simulink model "simulare_regulator_discret_etapa1"  (R2020a)
settings: Solver=VariableStepAuto  StartTime=0.0  StopTime=500  RelTol=1e-3
settings Model: Creator=user  LastModifiedBy=user

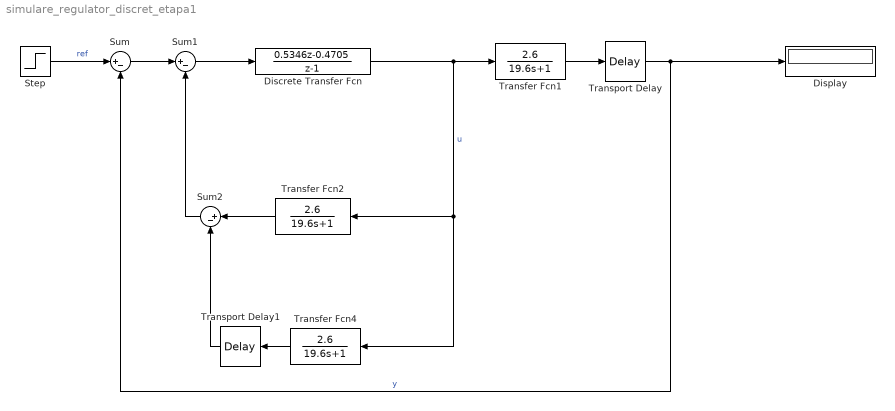
== system simulare_regulator_discret_etapa1 ==
  Discrete Transfer Fcn : DiscreteTransferFcn  Numerator=[0.5346 -0.4705]  Denominator=[1 -1]  SampleTime=2.5
  Display : Display
  Step : Step  SampleTime=2.5
  Sum : Sum  Inputs=|+-
  Sum1 : Sum  Inputs=|+-
  Sum2 : Sum  Inputs=|+-
  Transfer Fcn1 : TransferFcn  Numerator=[2.6]  Denominator=[19.6 1]
  Transfer Fcn2 : TransferFcn  Numerator=[2.6]  Denominator=[19.6 1]
  Transfer Fcn4 : TransferFcn  Numerator=[2.6]  Denominator=[19.6 1]
  Transport Delay : TransportDelay  DelayTime=5
  Transport Delay1 : TransportDelay  DelayTime=5
  wires:
  Transport Delay1/1 -> Sum2/2
  Sum2/1 -> Sum1/2
  Transfer Fcn4/1 -> Transport Delay1/1
  Transport Delay/1 -> Display/1, Sum/2  "y"
  Sum/1 -> Sum1/1
  Transfer Fcn2/1 -> Sum2/1
  Step/1 -> Sum/1  "ref"
  Transfer Fcn1/1 -> Transport Delay/1
  Sum1/1 -> Discrete Transfer Fcn/1
  Discrete Transfer Fcn/1 -> Transfer Fcn4/1, Transfer Fcn2/1, Transfer Fcn1/1  "u"
